simulink model "Rider_Controls_InHardware"  (R2014b)
settings: configuration reference "Embedded_Configuration" (kept outside this file)
PostLoadFcn:
  | load('Embedded_Config.mat')
model workspace: external: MAT-File Rider_Controls_InHardware.mat (data not in the file)
undefined symbols (not defined in the file or in its folder): alpha
libraries: c2802xlib x1, canmsglib x1, c2803xlib x1, c280xlib x1
settings Model: Creator=The MathWorks Inc.  LastModifiedBy=Sean

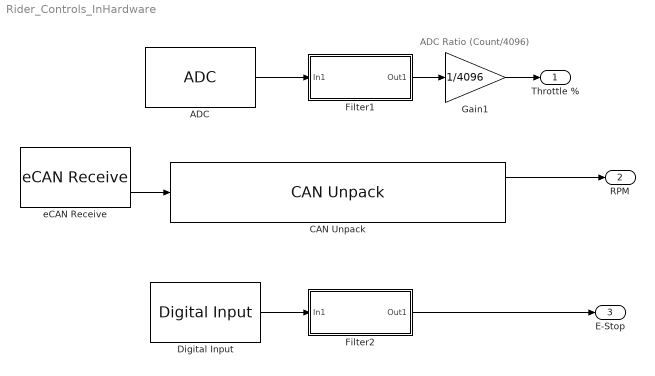
== system Rider_Controls_InHardware ==
  note: ADC Ratio (Count/4096)
  ADC : c2802xlib/ADC  ADCModule=1  samplingMode=Single sample mode  useSOC1=SOC0  useSOC2=SOC0_SOC1  SOCAcquisitionWindow=7  SOCTriggerSource=Software  SOCInterruptTrigger=No ADCINT  Ts=0.00001  dType=single  postInterrupt=off  interruptSel=ADCINT1  ADCINTContinuous=off  endma=off  chdma=1  conv1=ADCINA7  conv2=ADCINA0 and ADCINB0
  CAN Unpack : canmsglib/CAN Unpack  CANdbFile=C:\Users\Nathan\Desktop\Git\Databases\RW3.dbc  MsgList=Velocity_Measurement  MsgName=Velocity_Measurement  MsgIDType=Standard (11-bit identifier)  MsgIdentifier=1027  MsgLength=8  SignalInfo=Motor_Velocity$0$32$1$3$1$0$1$0$-Inf$Inf$#Vehicle_Velocity$32$32$1$3$1$0$1$0$-Inf$Inf$#  NSignals=2  IDPort=off  TimestampPort=off  ErrorPort=off  RemotePort=off  LengthPort=off  StatusPort=off  StartBits=str2num('[int32(0);int32(32)]')  SignalSizes=str2num('[int32(32);int32(32)]')  ByteOrders=str2num('[int32(1);int32(1)]')  DataTypes=str2num('[int32(3);int32(3)]')  MultiplexTypes=str2num('[int32(1);int32(1)]')  MultiplexValues=str2num('[double(0);double(0)]')  Factors=str2num('[double(1);double(1)]')  Offsets=str2num('[double(0);double(0)]')  Minimums=str2num('[double(-Inf);double(-Inf)]')  Maximums=str2num('[double(Inf);double(Inf)]')
      settings: DataFormat=CANdb specified signals
  Digital Input : c2803xlib/Digital Input  GPIO_Number=GPIO24~GPIO31  GPIO_Bit0=off  GPIO_Bit1=off  GPIO_Bit2=on  GPIO_Bit3=off  GPIO_Bit4=off  GPIO_Bit5=off  GPIO_Bit6=off  GPIO_Bit7=off  sampleTime=0.001  dataType=auto  GPIO_Bit0_Qualification=Sync to SYSCLKOUT  GPIO_Bit1_Qualification=Sync to SYSCLKOUT  GPIO_Bit2_Qualification=Sync to SYSCLKOUT  GPIO_Bit3_Qualification=Sync to SYSCLKOUT  GPIO_Bit4_Qualification=Sync to SYSCLKOUT  GPIO_Bit5_Qualification=Sync to SYSCLKOUT  GPIO_Bit6_Qualification=Sync to SYSCLKOUT  GPIO_Bit7_Qualification=Sync to SYSCLKOUT  Qualification_Period=-1
  Filter1 : Subsystem
  Filter2 : Subsystem
  Gain1 : Gain  Gain=1/4096  OutDataTypeStr=single
  eCAN Receive : c280xlib/eCAN Receive  chipFamily=C280x  useModule=eCAN_A  mailboxNo=2  messageID=1027  messageType=Standard (11-bit identifier)  sampleTime=.01  dataType=CAN_MESSAGE_TYPE  initValue=0  outputMessageLength=off  outputMessageTimeStamp=off  postInterrupt=off  interruptLine=0
  Throttle % : Outport  OutDataTypeStr=single
  RPM : Outport  Port=2  OutDataTypeStr=single  SampleTime=.01
  E-Stop : Outport  Port=3
  wires:
  eCAN Receive/2 -> CAN Unpack/1
  CAN Unpack/1 -> RPM/1
  Filter1/1(Out1) -> Gain1/1
  ADC/1 -> Filter1/1(In1)
  Gain1/1 -> Throttle %/1
  Digital Input/1 -> Filter2/1(In1)
  Filter2/1(Out1) -> E-Stop/1

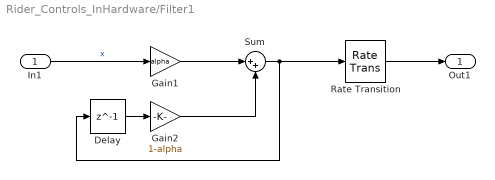
== system Rider_Controls_InHardware/Filter1 ==
  In1 : Inport
  Delay : Delay  DelayLength=1
  Gain1 : Gain  Gain=alpha
  Gain2 : Gain  Gain=1-alpha
  Rate Transition : RateTransition  OutPortSampleTime=.01
  Sum : Sum  Inputs=|++  OutDataTypeStr=single
  Out1 : Outport  SampleTime=.01
  wires:
  Rate Transition/1 -> Out1/1
  Sum/1 -> Delay/1, Rate Transition/1
  Gain2/1 -> Sum/2
  Delay/1 -> Gain2/1
  Gain1/1 -> Sum/1
  In1/1 -> Gain1/1  "x"

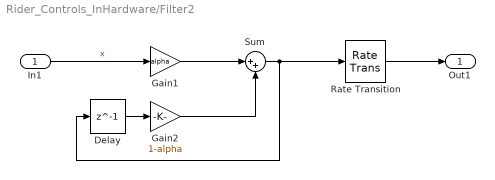
== system Rider_Controls_InHardware/Filter2 ==
  In1 : Inport
  Delay : Delay  DelayLength=1
  Gain1 : Gain  Gain=alpha
  Gain2 : Gain  Gain=1-alpha
  Rate Transition : RateTransition  OutPortSampleTime=.01
  Sum : Sum  Inputs=|++  OutDataTypeStr=single
  Out1 : Outport  SampleTime=.01
  wires:
  Rate Transition/1 -> Out1/1
  Sum/1 -> Delay/1, Rate Transition/1
  Gain2/1 -> Sum/2
  Delay/1 -> Gain2/1
  Gain1/1 -> Sum/1
  In1/1 -> Gain1/1  "x"
